simulink model "Control_model_matching_lineal"  (R2023a)
settings: Solver=FixedStepAuto  StartTime=0.0  StopTime=70  FixedStep=Ts  RelTol=1e-3
values from neighbouring files (symbols this model uses):
  Ts = 0.001    [DatosSimulador.mat]
  TsMot = 0.001    [DatosSimulador.mat]
  TsPos = 0.002    [DatosSimulador.mat]
  TsRef = 0.02    [DatosSimulador.mat]
  TsSenF = 0.001    [DatosSimulador.mat]
  TsVel = 0.001    [DatosSimulador.mat]
undefined symbols (not defined in the file or in its folder): denC2, denG, denM, denPitch, denRoll, FC, NP, numC2, numG, numM, numPitch, numRoll, uo
libraries: simulink x2
(part 2 of 2)

== matlab function Control_model_matching_lineal/Modelo UAV lineal/Dinamica UAV/Rotacion ==
  settings: updateMethod=DISCRETE
  data: Q output; Wb input size=3; Euler output size=3; Tiempo input
function [Q, Euler] = RotacionAngular(Wb, Tiempo)

persistent q TiempoAnterior

if isempty(q)
    q  = [1 0 0 0];
    TiempoAnterior = 0;
end

dt = Tiempo - TiempoAnterior;
TiempoAnterior = Tiempo;

W = [0 0 0]';
Euler = [0 0 0]';

% Se integra la tasa de cambio de cuaternion
W(1) = Wb(1) * (0.5 * dt);
W(2) = Wb(2) * (0.5 * dt);
W(3) = Wb(3) * (0.5 * dt);

q1 = q(1);
q2 = q(2);
q3 = q(3);

q(1) = q(1) + (-q2 * W(1) - q3 * W(2) - q(4) * W(3));
q(2) = q(2) + ( q1 * W(1) + q3 * W(3) - q(4) * W(2));
q(3) = q(3) + ( q1 * W(2) - q2 * W(3) + q(4) * W(1));
q(4) = q(4) + ( q1 * W(3) + q2 * W(2) - q3   * W(1));


% Se normaliza el cuaternion
Q = q / norm(q);

% Ecuaciones sacadas de Madgwick con el conjugado implicito en las formulas
Euler(1) = atan2(2 * Q(3) * Q(4) + 2 * Q(1) * Q(2), 2 * Q(1) * Q(1) + 2 * Q(4) * Q(4) - 1);
Euler(2) = -asin(2 * (Q(2) * Q(4) - Q(1) * Q(3)));
Euler(3) = atan2(2 * Q(2) * Q(3) + 2 * Q(1) * Q(4), 2 * Q(1) * Q(1) + 2 * Q(2) * Q(2) - 1);

== matlab function Control_model_matching_lineal/Estimacion lineal/Filtro pasa bajos  acelerometro/MATLAB Function1 ==
  settings: updateMethod=DISCRETE
  data: In input; Fc input; Out output; Ts input
function Out  = LowPassFilterP2(In, Fc, Ts)

persistent b0 b1 b2 a1 a2 a0 in1 in2 out1 out2

if isempty(b0)
    ohm     = 2 * pi * Fc;
    damping = 1 / (sqrt(2));

    b2 = Ts^2 * ohm^2;
    b1 = 2.0 * b2;
    b0 = b2;

    a2 = 4.0 + 4.0 * damping * ohm * Ts + b2;
    a1 = -8.0 + b1;
    a0 = 4.0 - 4.0 * damping * ohm * Ts + b2;

    in1  = 0;
    in2  = 0;
    out1 = 0;
    out2 = 0;
end

Out = (b2 * In + b1 * in1 + b0 * in2 - a1 * out1 - a0 * out2) / a2;

in2  = in1;
in1  = In;
out2 = out1;
out1 = Out;

== matlab function Control_model_matching_lineal/Estimacion lineal/Filtro pasa bajos  acelerometro/MATLAB Function2 ==
  settings: updateMethod=DISCRETE
  data: In input; Fc input; Out output; Ts input
function Out  = LowPassFilterP2(In, Fc, Ts)

persistent b0 b1 b2 a1 a2 a0 in1 in2 out1 out2

if isempty(b0)
    ohm     = 2 * pi * Fc;
    damping = 1 / (sqrt(2));

    b2 = Ts^2 * ohm^2;
    b1 = 2.0 * b2;
    b0 = b2;

    a2 = 4.0 + 4.0 * damping * ohm * Ts + b2;
    a1 = -8.0 + b1;
    a0 = 4.0 - 4.0 * damping * ohm * Ts + b2;

    in1  = 0;
    in2  = 0;
    out1 = 0;
    out2 = 0;
end

Out = (b2 * In + b1 * in1 + b0 * in2 - a1 * out1 - a0 * out2) / a2;

in2  = in1;
in1  = In;
out2 = out1;
out1 = Out;

== matlab function Control_model_matching_lineal/Estimacion lineal/Filtro pasa bajos  acelerometro/MATLAB Function3 ==
  settings: updateMethod=DISCRETE
  data: In input; Fc input; Out output; Ts input
function Out  = LowPassFilterP1(In, Fc, Ts)

persistent b0 b1 a0 a1 in1 out1

if isempty(b0)
    ohm = 2.0 * pi * Fc;

    b1 = ohm * Ts;
    b0 = b1;
    a1 = 2.0 + b1;
    a0 = b1 - 2.0;

    in1  = 0;
    out1 = 0;
end

Out = (b1 * In + b0 * in1 - a0 * out1) / a1;

in1  = In;
out1 = Out;
